simulink model "BatteryStoragePVPlantGFM"  (R2023a)
settings: Solver=FixedStepDiscrete  StartTime=0.0  StopTime=SimulationTime  RelTol=1e-3
PreLoadFcn:
  | run('BatteryStoragePVPlantGFMParameters')
undefined symbols (not defined in the file): Array, Base, battery, BatteryInverter, DiscIntNeverNeededParam, ee, Feeder, fRT, GFLBatteryController, GFMBatteryController, Grid, GridTransformer, Line, Load, Load2CB_final, Load2CB_initial, LVRT, maxSoC, maxVdc, minIrrad, minSoC, minVdc, Mpp, olTime, Panel, PVController, PVInverter, PVTransformer, Scenario, SM, SubTransmissionLine, Ts, VSMbase
libraries: ee_lib x51, nesl_utility x45, fl_lib x26, eeGeneralControl x18, simulink x12, eeTransforms x11, slpidlib x8, eePowerMeasurement x5, batteryecm_lib x2, eeTotalHarmonicDistorsion x2, spsLeadLagFilterLib x1, eeSmAC1C x1
(part 4 of 5)

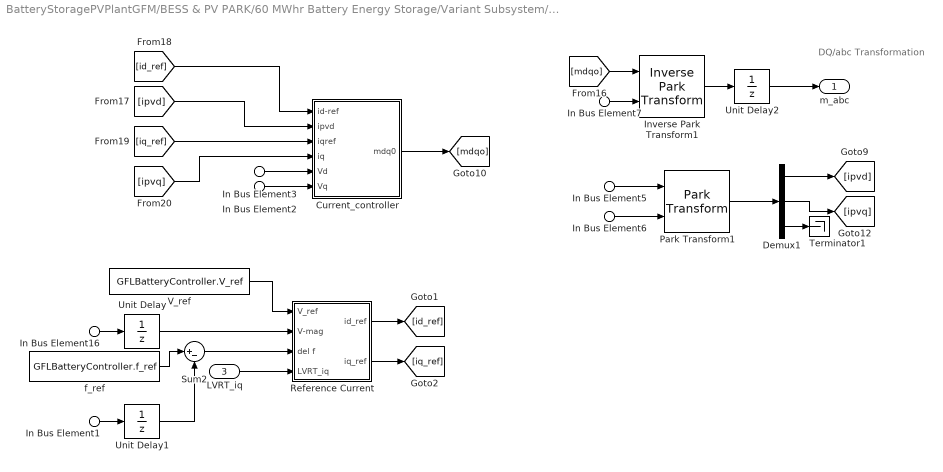
== system BatteryStoragePVPlantGFM/BESS & PV PARK/60 MWhr Battery Energy Storage/Variant Subsystem/Grid Following Support/Battery Inverter/GFL Battery Controller ==
  note: DQ/abc Transformation
  In Bus Element3 : Inport  PortName=Vbus  Element=Vd
  In Bus Element16 : Inport  PortName=Vbus  Element=Vd
  In Bus Element2 : Inport  PortName=Vbus  Element=Vq
  In Bus Element6 : Inport  PortName=Vbus  Element=Theta
  In Bus Element7 : Inport  PortName=Vbus  Element=Theta
  In Bus Element1 : Inport  PortName=Vbus  Element=w
  In Bus Element5 : Inport  Port=2  PortName=ipv2  Element=1
  LVRT_iq : Inport  Port=3
  Current_controller : Subsystem
  Demux1 : Demux  Outputs=3
  Inverse Park Transform1 : eeTransforms/Inverse Park Transform  AxisAlignment=Q-axis  PowerInvariant=off
  Park Transform1 : eeTransforms/Park Transform  AxisAlignment=Q-axis  PowerInvariant=off
  Reference Current : Subsystem
  Sum2 : Sum  Inputs=|+-
  Terminator1 : Terminator
  Unit Delay : UnitDelay  SampleTime=GFLBatteryController.Td  HasFrameUpgradeWarning=on
  Unit Delay1 : UnitDelay  SampleTime=GFLBatteryController.Td  HasFrameUpgradeWarning=on
  Unit Delay2 : UnitDelay  SampleTime=Ts  HasFrameUpgradeWarning=on
  V_ref : Constant  Value=GFLBatteryController.V_ref
  f_ref : Constant  Value=GFLBatteryController.f_ref
  m_abc : Outport
  wires:
  In Bus Element2/1 -> Current_controller/6(Vq)
  Current_controller/1(mdq0) -> [mdqo]
  Inverse Park Transform1/1 -> Unit Delay2/1
  Demux1/2 -> [ipvq]
  Unit Delay2/1 -> m_abc/1
  Demux1/1 -> [ipvd]
  Demux1/3 -> Terminator1/1
  [mdqo] -> Inverse Park Transform1/1
  Park Transform1/1 -> Demux1/1
  [id_ref] -> Current_controller/1(id-ref)
  In Bus Element3/1 -> Current_controller/5(Vd)
  [iq_ref] -> Current_controller/3(iqref)
  [ipvq] -> Current_controller/4(iq)
  In Bus Element6/1 -> Park Transform1/2
  In Bus Element7/1 -> Inverse Park Transform1/2
  [ipvd] -> Current_controller/2(ipvd)
  In Bus Element5/1 -> Park Transform1/1
  f_ref/1 -> Sum2/1
  V_ref/1 -> Reference Current/1(V_ref)
  In Bus Element16/1 -> Unit Delay/1
  LVRT_iq/1 -> Reference Current/4(LVRT_iq)
  Sum2/1 -> Reference Current/3(del f)
  Reference Current/2(iq_ref) -> [iq_ref]
  Reference Current/1(id_ref) -> [id_ref]
  In Bus Element1/1 -> Unit Delay1/1
  Unit Delay1/1 -> Sum2/2
  Unit Delay/1 -> Reference Current/2(V-mag)

== system BatteryStoragePVPlantGFM/BESS & PV PARK/60 MWhr Battery Energy Storage/Variant Subsystem/Grid Following Support/Battery Inverter/Inverter ==
  m_abc : Inport
  Average-Value Voltage Source Converter (Three-Phase) : ee_lib/Semiconductors & Converters/Converters/Average-Value Voltage Source Converter (Three-Phase)  port_option=ee.enum.threePhasePort.composite  frequency_option=ee.enum.converters.frequency.variable  FRated=60 Hz  losses_parameterization=ee.enum.converters.losses.fixed  Pfixed=1 W  ks=0.01  kc1=1.7 V  kc2=0.01 Ohm  Ploss_vect=[100, 800, 1870, 3250, 4900] W  Irms_vect=[10, 100, 200, 300, 400] A  Vdc_nom=300 V  thermal_mass=30000 J/K  temperature_specify=off  temperature_priority=High  temperature=298.15 K  temperature_nominal_specify=off  temperature_nominal_unit=K  temperature_nominal_value=1
      settings: InternalSimscapePortConfiguration="{\"Bottom\":[],\"Left\":[{\"id\":\"ModWave\",\"label\":\"ModWave\",\"type\":\"input\"},{\"id\":\"N\",\"label\":\"~\",\"type\":\"foundation.electrical.three_phase\"}],\"Right\":[{\"id\":\"p\",\"label\":\"+\",\"type\":\"foundation.electrical.electrical\"},{\"id\":\"n\",\"label\":\"-\",\"type\":\"foundation.electrical.electrical\"}],\"Top\":[]}"
  Average-Value DC-DC Converter : ee_lib/Semiconductors & Converters/Converters/Average-Value DC-DC Converter  control_option=ee.enum.converters.controlinput.voltage  converter_type=ee.enum.converters.dcdctype.buckboost  efficiency_option=ee.enum.converters.efficiency.constant  efficiency_fixed=99  i_vec=[0, 2, 5] A  efficiency_vec=[90, 95, 98]
      settings: InternalSimscapePortConfiguration="{\"Bottom\":[],\"Left\":[{\"id\":\"Vref\",\"label\":\"Vref\",\"type\":\"input\"},{\"id\":\"p1\",\"label\":\"1+\",\"type\":\"foundation.electrical.electrical\"},{\"id\":\"n1\",\"label\":\"1-\",\"type\":\"foundation.electrical.electrical\"}],\"Right\":[{\"id\":\"p2\",\"label\":\"2+\",\"type\":\"foundation.electrical.electrical\"},{\"id\":\"n2\",\"label\":\"2-\",\"type\":\"foundation.electrical.electrical\"}],\"Top\":[]}"
  Capacitor : fl_lib/Electrical/Electrical Elements/Capacitor  c=GFMBatteryController.C_dc F  r=1e-6 Ohm  g=0 1/Ohm  i_specify=off  i_priority=None  i=0 A  i_nominal_specify=off  i_nominal_unit=A  i_nominal_value=1  v_specify=off  v_priority=None  v=6560*.5 V  v_nominal_specify=off  v_nominal_unit=V  v_nominal_value=1  vc_specify=on  vc_priority=None  vc=PVInverter.Vdc V  vc_nominal_specify=off  vc_nominal_unit=V  vc_nominal_value=1
  Constant : Constant  Value=PVInverter.Vdc
  ERef1 : fl_lib/Electrical/Electrical Elements/Electrical Reference
  PS-Simulink Converter : nesl_utility/PS-Simulink Converter  PhysicalDomain=network_engine_domain  SubClassName=ps_output  LeftPortType=input  RightPortType=output  PseudoPeriodic=off  Frequencies=[]  VectorFormat=inherit  Unit=inherit  AffineConversion=off
  Simulink-PS Converter2 : nesl_utility/Simulink-PS Converter  PhysicalDomain=network_engine_domain  SubClassName=ps_input  LeftPortType=input  RightPortType=output  PseudoPeriodic=off  Frequencies=[]  NoiseDistribution=none  NoiseParameters=[]  Unit=1  AffineConversion=off  FilteringAndDerivatives=provide  SimscapeFilterOrder=1  InputFilterTimeConstant=0.001  UdotUserProvided=0
  Simulink-PS Converter3 : nesl_utility/Simulink-PS Converter  PhysicalDomain=network_engine_domain  SubClassName=ps_input  LeftPortType=input  RightPortType=output  PseudoPeriodic=off  Frequencies=[]  NoiseDistribution=none  NoiseParameters=[]  Unit=1  AffineConversion=off  FilteringAndDerivatives=provide  SimscapeFilterOrder=1  InputFilterTimeConstant=0.001  UdotUserProvided=0
  Unit Delay : UnitDelay  SampleTime=-1  HasFrameUpgradeWarning=on
  Voltage Sensor : fl_lib/Electrical/Electrical Sensors/Voltage Sensor
  battery : batteryecm_lib/Battery  Vnom=battery.vbat_nominal V  prm_dir=simscape.enum.battery.prm_dir.disabled  R1_dis=2 Ohm  R1_ch=2 Ohm  R1=battery.resistance Ohm  prm_AH=simscape.enum.battery.prm_AH.finite  AH=battery.capacity A*hr  V1=battery.vbat_1 V  AH1=battery.charge_vbat1 A*hr  prm_R2=simscape.enum.battery.prm_R2.disabled  R2=2000 Ohm  Tmeas=298.15 K  charge_measurement_port=simscape.enum.battery.enable.no  prm_dyn=simscape.enum.battery.prm_dyn.off  Rp1=0.005 Ohm  tau1=30 s  Rp2=0.005 Ohm  tau2=30 s  Rp3=0.005 Ohm  tau3=30 s  Rp4=0.005 Ohm  tau4=30 s  Rp5=0.005 Ohm  tau5=30 s  prm_fade=simscape.enum.battery.prm_fade.disabled  N_fade=100  AH_fade=45 A*hr  R1_fade=2.02 Ohm  R1_ch_fade=2.02 Ohm  V1_fade=10.35 V  prm_age=simscape.enum.battery.prm_age.disabled  prm_age_OCV=simscape.enum.battery.prm_age_OCV.OCV  OCV_age=0.9  SOC_age=60  Tmeas_age=298.15 K  delta_time_age_vec=[0] d  temperature_age_vec=[273] K  OCV_scaling_age=2.2134e6  OCV_offset_age=1.632e6  temp_exp_age=0.515833569 V  t_exp_age=0.75  Vnom_T2=12 V  R1_T2=2.2 Ohm  R1_T2_dis=2.2 Ohm  R1_T2_ch=2.2 Ohm  V1_T2=11.4 V  R2_T2=2200 Ohm  Rp1_T2=0.005 Ohm  tau1_T2=30 s  Rp2_T2=0.005 Ohm  tau2_T2=30 s  Rp3_T2=0.005 Ohm  tau3_T2=30 s  Rp4_T2=0.005 Ohm  tau4_T2=30 s  Rp5_T2=0.005 Ohm  tau5_T2=30 s  Tmeas2=273.15 K  thermal_port=simscape.enum.thermaleffects.omit  thermal_mass=30000 J/K  i_specify=off  i_priority=None  i=0 A  i_nominal_specify=off  i_nominal_unit=A  i_nominal_value=1  v_specify=on  v_priority=None  v=6000 V  v_nominal_specify=off  v_nominal_unit=V  v_nominal_value=1  charge_specify=off  charge_priority=High  charge=50 A*hr  charge_nominal_specify=off  charge_nominal_unit=A*hr  charge_nominal_value=1  num_cycles_specify=off  num_cycles_priority=High  num_cycles=0  num_cycles_nominal_specify=off  num_cycles_nominal_unit=1  num_cycles_nominal_value=1  temperature_specify=off  temperature_priority=High  temperature=298.15 K  temperature_nominal_specify=off  temperature_nominal_unit=K  temperature_nominal_value=1
  abc : PMIOPort  Side=Right
  wires:
  Constant/1 -> Unit Delay/1
  Unit Delay/1 -> Simulink-PS Converter3/1
  m_abc/1 -> Simulink-PS Converter2/1
  PS-Simulink Converter/1 -> [Vdc]
  connections:
  Average-Value DC-DC Converter/RConn2 -- ERef1/LConn1 -- Capacitor/RConn1 -- Average-Value Voltage Source Converter (Three-Phase)/RConn2 -- Voltage Sensor/RConn2
  Average-Value DC-DC Converter/RConn1 -- Capacitor/LConn1 -- Average-Value Voltage Source Converter (Three-Phase)/RConn1 -- Voltage Sensor/LConn1
  Simulink-PS Converter3/RConn1 -- Average-Value DC-DC Converter/LConn1
  Average-Value Voltage Source Converter (Three-Phase)/LConn1 -- Simulink-PS Converter2/RConn1
  battery/RConn1 -- Average-Value DC-DC Converter/LConn3
  battery/LConn1 -- Average-Value DC-DC Converter/LConn2
  PS-Simulink Converter/LConn1 -- Voltage Sensor/RConn1
  abc/RConn1 -- Average-Value Voltage Source Converter (Three-Phase)/LConn2

== system BatteryStoragePVPlantGFM/BESS & PV PARK/60 MWhr Battery Energy Storage/Variant Subsystem/Grid Forming VSM/Battery Inverter B1/Inverter ==
  note: DC bus voltage reference
  reference : Inport
  "Average DC_DC bidirectional Converter " : ee_lib/Semiconductors & Converters/Converters/Average-Value DC-DC Converter  control_option=ee.enum.converters.controlinput.voltage  converter_type=ee.enum.converters.dcdctype.buckboost  efficiency_option=ee.enum.converters.efficiency.constant  efficiency_fixed=99  i_vec=[0, 2, 5] A  efficiency_vec=[90, 95, 98]
      settings: InternalSimscapePortConfiguration="{\"Bottom\":[],\"Left\":[{\"id\":\"Vref\",\"label\":\"Vref\",\"type\":\"input\"},{\"id\":\"p1\",\"label\":\"1+\",\"type\":\"foundation.electrical.electrical\"},{\"id\":\"n1\",\"label\":\"1-\",\"type\":\"foundation.electrical.electrical\"}],\"Right\":[{\"id\":\"p2\",\"label\":\"2+\",\"type\":\"foundation.electrical.electrical\"},{\"id\":\"n2\",\"label\":\"2-\",\"type\":\"foundation.electrical.electrical\"}],\"Top\":[]}"
  Average-Value Voltage Source Inverter : ee_lib/Semiconductors & Converters/Converters/Average-Value Voltage Source Converter (Three-Phase)  port_option=ee.enum.threePhasePort.composite  frequency_option=ee.enum.converters.frequency.variable  FRated=60 Hz  losses_parameterization=ee.enum.converters.losses.fixed  Pfixed=0.1 W  ks=0.01  kc1=1.7 V  kc2=0.01 Ohm  Ploss_vect=[100, 800, 1870, 3250, 4900] W  Irms_vect=[10, 100, 200, 300, 400] A  Vdc_nom=300 V  thermal_mass=30000 J/K  temperature_specify=off  temperature_priority=High  temperature=298.15 K  temperature_nominal_specify=off  temperature_nominal_unit=K  temperature_nominal_value=1
      settings: InternalSimscapePortConfiguration="{\"Bottom\":[],\"Left\":[{\"id\":\"ModWave\",\"label\":\"ModWave\",\"type\":\"input\"},{\"id\":\"N\",\"label\":\"~\",\"type\":\"foundation.electrical.three_phase\"}],\"Right\":[{\"id\":\"p\",\"label\":\"+\",\"type\":\"foundation.electrical.electrical\"},{\"id\":\"n\",\"label\":\"-\",\"type\":\"foundation.electrical.electrical\"}],\"Top\":[]}"
  Battery (60MWhr) : batteryecm_lib/Battery  Vnom=battery.vbat_nominal V  prm_dir=simscape.enum.battery.prm_dir.disabled  R1_dis=2 Ohm  R1_ch=2 Ohm  R1=battery.resistance Ohm  prm_AH=simscape.enum.battery.prm_AH.finite  AH=battery.capacity A*hr  V1=battery.vbat_1 V  AH1=battery.charge_vbat1 A*hr  prm_R2=simscape.enum.battery.prm_R2.disabled  R2=2000 Ohm  Tmeas=298.15 K  charge_measurement_port=simscape.enum.battery.enable.no  prm_dyn=simscape.enum.battery.prm_dyn.off  Rp1=0.005 Ohm  tau1=30 s  Rp2=0.005 Ohm  tau2=30 s  Rp3=0.005 Ohm  tau3=30 s  Rp4=0.005 Ohm  tau4=30 s  Rp5=0.005 Ohm  tau5=30 s  prm_fade=simscape.enum.battery.prm_fade.disabled  N_fade=100  AH_fade=45 A*hr  R1_fade=2.02 Ohm  R1_ch_fade=2.02 Ohm  V1_fade=10.35 V  prm_age=simscape.enum.battery.prm_age.disabled  prm_age_OCV=simscape.enum.battery.prm_age_OCV.OCV  OCV_age=0.9  SOC_age=60  Tmeas_age=298.15 K  delta_time_age_vec=[0] d  temperature_age_vec=[273] K  OCV_scaling_age=2.2134e6  OCV_offset_age=1.632e6  temp_exp_age=0.515833569 V  t_exp_age=0.75  Vnom_T2=12 V  R1_T2=2.2 Ohm  R1_T2_dis=2.2 Ohm  R1_T2_ch=2.2 Ohm  V1_T2=11.4 V  R2_T2=2200 Ohm  Rp1_T2=0.005 Ohm  tau1_T2=30 s  Rp2_T2=0.005 Ohm  tau2_T2=30 s  Rp3_T2=0.005 Ohm  tau3_T2=30 s  Rp4_T2=0.005 Ohm  tau4_T2=30 s  Rp5_T2=0.005 Ohm  tau5_T2=30 s  Tmeas2=273.15 K  thermal_port=simscape.enum.thermaleffects.omit  thermal_mass=30000 J/K  i_specify=off  i_priority=None  i=0 A  i_nominal_specify=off  i_nominal_unit=A  i_nominal_value=1  v_specify=on  v_priority=None  v=6000 V  v_nominal_specify=off  v_nominal_unit=V  v_nominal_value=1  charge_specify=off  charge_priority=High  charge=50 A*hr  charge_nominal_specify=off  charge_nominal_unit=A*hr  charge_nominal_value=1  num_cycles_specify=off  num_cycles_priority=High  num_cycles=0  num_cycles_nominal_specify=off  num_cycles_nominal_unit=1  num_cycles_nominal_value=1  temperature_specify=off  temperature_priority=High  temperature=298.15 K  temperature_nominal_specify=off  temperature_nominal_unit=K  temperature_nominal_value=1
  Capacitor : fl_lib/Electrical/Electrical Elements/Capacitor  c=GFMBatteryController.C_dc F  r=1e-6 Ohm  g=0 1/Ohm  i_specify=off  i_priority=None  i=0 A  i_nominal_specify=off  i_nominal_unit=A  i_nominal_value=1  v_specify=off  v_priority=None  v=6560*.5 V  v_nominal_specify=off  v_nominal_unit=V  v_nominal_value=1  vc_specify=on  vc_priority=None  vc=PVInverter.Vdc V  vc_nominal_specify=off  vc_nominal_unit=V  vc_nominal_value=1
  Constant : Constant  Value=PVInverter.Vdc
  ERef1 : fl_lib/Electrical/Electrical Elements/Electrical Reference
  PS-Simulink Converter : nesl_utility/PS-Simulink Converter  PhysicalDomain=network_engine_domain  SubClassName=ps_output  LeftPortType=input  RightPortType=output  PseudoPeriodic=off  Frequencies=[]  VectorFormat=inherit  Unit=inherit  AffineConversion=off
  Simulink-PS Converter2 : nesl_utility/Simulink-PS Converter  PhysicalDomain=network_engine_domain  SubClassName=ps_input  LeftPortType=input  RightPortType=output  PseudoPeriodic=off  Frequencies=[]  NoiseDistribution=none  NoiseParameters=[]  Unit=1  AffineConversion=off  FilteringAndDerivatives=provide  SimscapeFilterOrder=1  InputFilterTimeConstant=0.001  UdotUserProvided=0
  Simulink-PS Converter3 : nesl_utility/Simulink-PS Converter  PhysicalDomain=network_engine_domain  SubClassName=ps_input  LeftPortType=input  RightPortType=output  PseudoPeriodic=off  Frequencies=[]  NoiseDistribution=none  NoiseParameters=[]  Unit=1  AffineConversion=off  FilteringAndDerivatives=provide  SimscapeFilterOrder=1  InputFilterTimeConstant=0.001  UdotUserProvided=0
  Unit Delay : UnitDelay  SampleTime=-1  HasFrameUpgradeWarning=on
  Voltage Sensor : fl_lib/Electrical/Electrical Sensors/Voltage Sensor
  abc : PMIOPort  Side=Right
  wires:
  PS-Simulink Converter/1 -> [Vdc]
  reference/1 -> Simulink-PS Converter2/1
  Unit Delay/1 -> Simulink-PS Converter3/1
  Constant/1 -> Unit Delay/1
  connections:
  PS-Simulink Converter/LConn1 -- Voltage Sensor/RConn1
  Capacitor/LConn1 -- Average-Value Voltage Source Inverter/RConn1 -- "Average DC_DC bidirectional Converter "/RConn1 -- Voltage Sensor/LConn1
  ERef1/LConn1 -- Capacitor/RConn1 -- Average-Value Voltage Source Inverter/RConn2 -- Voltage Sensor/RConn2 -- "Average DC_DC bidirectional Converter "/RConn2
  Average-Value Voltage Source Inverter/LConn1 -- Simulink-PS Converter2/RConn1
  abc/RConn1 -- Average-Value Voltage Source Inverter/LConn2
  Simulink-PS Converter3/RConn1 -- "Average DC_DC bidirectional Converter "/LConn1
  Battery (60MWhr)/LConn1 -- "Average DC_DC bidirectional Converter "/LConn2
  Battery (60MWhr)/RConn1 -- "Average DC_DC bidirectional Converter "/LConn3

== system BatteryStoragePVPlantGFM/BESS & PV PARK/60 MWhr Battery Energy Storage/Variant Subsystem/Grid Forming VSM/Battery Inverter B1/controller ==
  In Bus Element : Inport  PortName=Bat  Element=Iabc_bat
  In Bus Element1 : Inport  PortName=Bat  Element=Vabc_bat
  Constant : Constant  Value=GFMBatteryController.P_ref  SampleTime=Ts
  Constant1 : Constant  Value=GFMBatteryController.Q_ref  SampleTime=Ts
  GridFormingController : Subsystem  mask{power=VSMbase.power*1e3, girdLineVoltage=VSMbase.lineVoltage, powerFreq=VSMbase.frequency, powerControl=Virtual Synchronous Machine, activePowerSampleTime=GFMBatteryController.Sampletime, droopSlope=BatteryInverter.droopControl.freqSlopeMp, droopT1=BatteryInverter.droopControl.T1, droopT2=BatteryInverter.droopControl.T2, droopTC=BatteryInverter.droopControl.lpfTimeConst, vsmPmeasFilterTC=GFMBatteryController.filtertimeconstant, vsmFreqDroop=1/GFMBatteryController.frequencydroop, vsmInertiaTC=GFMBatteryController.VSMInertia, vsmDampingConst=GFMBatteryController.Damping, QVoltFilterTC=GFMBatteryController.reactivepowerfiltertimeconstant, QVoltDroop=GFMBatteryController.voltagedroop, currentLimit=Virtual Impedance, maxCurrentLimit=BatteryInverter.currentLimit.overNominalCurrent, ctLimitVirtualImp=BatteryInverter.currentLimit.virImpResistance, ctLimitXbyR=BatteryInverter.currentLimit.virImpXbyR, ctLimitMaxCurrent=BatteryInverter.currentLimit.currentIsdSaturationMax, ctLimitDelayTime=BatteryInverter.currentLimit.overCurrentIsdDelay, VdIGain=GFMBatteryController.voltagecontrolki, vdPGain=GFMBatteryController.voltagecontrolkp, voltControlTs=GFMBatteryController.voltagecontroltimeconstant, VdMaxCt=BatteryInverter.controller.VoltageMaxId, VdMinCt=BatteryInverter.controller.VoltageMinId, VqPGain=GFMBatteryController.voltagecontrolkp, VqIGain=GFMBatteryController.voltagecontrolki, VqMaxCt=BatteryInverter.controller.VoltageMaxIq, VqMinCt=BatteryInverter.controller.VoltageMinIq, dcBusVoltage=BatteryInverter.DCVoltage, filterInductance=BatteryInverter.L, currentControlTs=GFMBatteryController.currentcontrollersampletime, IdPGain=GFMBatteryController.currentcontrollerkp, IdIGain=GFMBatteryController.currentcontrollerki, IqPGain=GFMBatteryController.currentcontrollerkp, IqIGain=GFMBatteryController.currentcontrollerki}
      mask prompts: power "Gird power (kW)"; girdLineVoltage "Gird line voltage (V)"; powerFreq "Power frequency (Hz)"; powerControl "Active Power Control"; activePowerSampleTime "Sample time (s)"; droopSlope "Frequency droop slope (Hz/W)"; droopT1 "Lead-Lag Numerator time constant (s)"; droopT2 "Lead-Lag Denominator time constant (s)"; droopTC "Filter cut-off time constant (s)"; vsmPmeasFilterTC "P measurement filter time constant (s)"; vsmFreqDroop "Frequency droop gain"; vsmInertiaTC "Inertia time constant (s)"; vsmDampingConst "Damping constant (pu)"; QVoltFilterTC "Q measurement filter time constant (s)"; QVoltDroop "Voltage droop (pu)"; currentLimit "Current Limiting Method"; maxCurrentLimit "Current Limit (pu)"; ctLimitVirtualImp "Virtual impedance (pu)"; ctLimitXbyR "Virtual X/R ratio"; ctLimitMaxCurrent "Maximum allowed current (pu)"; ctLimitDelayTime "Max. current delay time (s)"; VdIGain "Vd integral gain"; vdPGain "Vd proportaion gain"; voltControlTs "Controller sample time (s)"; VdMaxCt "Vd max. current Limit (A)"; VdMinCt "Vd min. current Limit (A)"; VqPGain "Vq proportaion gain"; VqIGain "Vq integration gain"; VqMaxCt "Vq max. current Limit (A)"; VqMinCt "Vq min. current Limit (A)"; dcBusVoltage "DC bus voltage"; filterInductance "Filter inductance (H)"; currentControlTs "Controller sample time (s)"; IdPGain "Id proportaion gain"; IdIGain "Id integral gain"; IqPGain "Iq proportaion gain"; IqIGain "Iq integral gain"
      mask init:
      | powerChoice = get_param(gcb,'powerControl');
      | currentChoice = get_param(gcb,'currentLimit');
      | 
      | powerloc = [gcb, '/Power Control/ActivePowerControl']; 
      | currentloc = [gcb, '/Current Limiting/CurrentLimitingMethod'];
      | 
      | switch powerChoice
      |     case 'Virtual Synchronous Machine'
      |         set_param(powerloc, 'LabelModeActiveChoice', 'vsm');
      |     case 'Droop Control'
      |          set_param(powerloc, 'LabelModeActiveChoice', 'droop');
      |    otherwise
      |         disp('Choose proper active power control method')
      | end
      | switch currentChoice
      |     case 'Virtual Impedance'
      |           set_param(currentloc, 'LabelModeActiveChoice', 'virimp');
      |     case 'Current Limiting'
      |          set_param(currentloc, 'LabelModeActiveChoice', 'ctSat');
      |     case 'Both Virtual Impedance and Current Limiting'
      |             set_param(currentloc, 'LabelModeActiveChoice', 'both');
      |     otherwise
      |         disp('Choose proper current limiting method')
      | end
      mask TypeOptions powerControl: Virtual Synchronous Machine | Droop Control
      mask Callback powerControl:
      | h = Simulink.Mask.get(gcb);
      | slectedActivePowerControl=get_param(gcb,'powerControl');
      | %slectedActivePowerControl = h.Parameters(find(string({h.Parameters.Name}) == 'powerControl')).Value;
      | switch slectedActivePowerControl
      |     case 'Virtual Synchronous Machine'
      |         h.Parameters(find(string({h.Parameters.Name}) == 'droopSlope')).Visible = 'off';
      |         h.Parameters(find(string({h.Parameters.Name}) == 'droopTC')).Visible = 'off';
      |         h.Parameters(find(string({h.Parameters.Name}) == 'droopT1')).Visible = 'off';
      |         h.Parameters(find(string({h.Parameters.Name}) == 'droopT2')).Visible = 'off';
      |         h.Parameters(find(string({h.Parameters.Name}) == 'vsmPmeasFilterTC')).Visible = 'on';
      |         h.Parameters(find(string({h.Parameters.Name}) == 'vsmFreqDroop')).Visible = 'on';
      |         h.Parameters(find(string({h.Parameters.Name}) == 'vsmInertiaTC')).Visible = 'on';
      |         h.Parameters(find(string({h.Parameters.Name}) == 'vsmDampingConst')).Visible = 'on';
      |     case 'Droop Control'
      |         h.Parameters(find(string({h.Parameters.Name}) == 'droopSlope')).Visible = 'on';
      |         h.Parameters(find(string({h.Parameters.Name}) == 'droopTC')).Visible = 'on';
      |         h.Parameters(find(string({h.Parameters.Name}) == 'droopT1')).Visible = 'on';
      |         h.Parameters(find(string({h.Parameters.Name}) == 'droopT2')).Visible = 'on';
      |         h.Parameters(find(string({h.Parameters.Name}) == 'vsmPmeasFilterTC')).Visible = 'off';
      |         h.Parameters(find(string({h.Parameters.Name}) == 'vsmFreqDroop')).Visible = 'off';
      |         h.Parameters(find(string({h.Parameters.Name}) == 'vsmInertiaTC')).Visible = 'off';
      |         h.Parameters(find(string({h.Parameters.Name}) == 'vsmDampingConst')).Visible = 'off';
      |     otherwise
      |         disp('Choose proper active power control method')
      | end
      mask TypeOptions currentLimit: Virtual Impedance | Current Limiting
      mask Callback currentLimit:
      | currentLimit = 1;
      | h = Simulink.Mask.get(gcb);
      | currentLimitControl=get_param(gcb,'currentLimit');
      | %slectedActivePowerControl = h.Parameters(find(string({h.Parameters.Name}) == 'powerControl')).Value;
      | switch currentLimitControl
      |     case 'Virtual Impedance'
      |         h.Parameters(find(string({h.Parameters.Name}) == 'maxCurrentLimit')).Visible = 'on';
      |         h.Parameters(find(string({h.Parameters.Name}) == 'ctLimitVirtualImp')).Visible = 'on';
      |         h.Parameters(find(string({h.Parameters.Name}) == 'ctLimitXbyR')).Visible = 'on';
      |         h.Parameters(find(string({h.Parameters.Name}) == 'ctLimitMaxCurrent')).Visible = 'off';
      |         h.Parameters(find(string({h.Parameters.Name}) == 'ctLimitDelayTime')).Visible = 'off';
      |     case 'Current Limiting'
      |         h.Parameters(find(string({h.Parameters.Name}) == 'maxCurrentLimit')).Visible = 'off';
      |         h.Parameters(find(string({h.Parameters.Name}) == 'ctLimitVirtualImp')).Visible = 'off';
      |         h.Parameters(find(string({h.Parameters.Name}) == 'ctLimitXbyR')).Visible = 'off';
      |         h.Parameters(find(string({h.Parameters.Name}) == 'ctLimitMaxCurrent')).Visible = 'on';
      |         h.Parameters(find(string({h.Parameters.Name}) == 'ctLimitDelayTime')).Visible = 'on';
      |     case 'Both Virtual Impedance and Current Limiting'
      |         h.Parameters(find(string({h.Parameters.Name}) == 'maxCurrentLimit')).Visible = 'on';
      |         h.Parameters(find(string({h.Parameters.Name}) == 'ctLimitVirtualImp')).Visible = 'on';
      |         h.Parameters(find(string({h.Parameters.Name}) == 'ctLimitXbyR')).Visible = 'on';
      |         h.Parameters(find(string({h.Parameters.Name}) == 'ctLimitMaxCurrent')).Visible = 'on';
      |         h.Parameters(find(string({h.Parameters.Name}) == 'ctLimitDelayTime')).Visible = 'on';
      |     otherwise
      |         disp('Choose proper current limiting method')
      | end
      mask DialogControl Container8 Prompt: Grid-forming inverter parameters
      mask DialogControl Pcontrolgrp Prompt: Active Power Controller Parameters
      mask DialogControl QcontrolGrp Prompt: Reactive Power Controller Parameters
      mask DialogControl faultRideThroughGrp Prompt: Fault Ride Through Parameters
      mask DialogControl voltControlgrp Prompt: Voltage Controller Parameters
      mask DialogControl Container15currentContGrp Prompt: Current Controller Parameters
      mask Display: image('C:\Users\rajarshd\OneDrive - MathWorks\Simulation_Final\Pics\e_vsm.png'); % Use "Edit Image" on toolstrip to change.
  Unit Delay2 : UnitDelay  SampleTime=Ts  HasFrameUpgradeWarning=on
  mabc : Outport
  wires:
  GridFormingController/2(Pmeas) -> [Pmeas]
  GridFormingController/3(Qmeas) -> [Qmeas]
  Constant1/1 -> GridFormingController/2(Qref)
  GridFormingController/1(mabc) -> Unit Delay2/1
  Constant/1 -> GridFormingController/1(Pref)
  Unit Delay2/1 -> mabc/1
  In Bus Element/1 -> GridFormingController/3(Igabc)
  In Bus Element1/1 -> GridFormingController/4(Vgabc)

== system BatteryStoragePVPlantGFM/BESS & PV PARK/100 MWp PV Park/PV Inverter A1/PV Controller/DC voltage controller & current reference/Subsystem1/V_dc_Controller1 ==
  PV_plant1 : Inport
  In2 : Inport  Port=2
  Gain : Gain  Gain=1/PVController.Vdc_base
  PID Controller : slpidlib/PID Controller  Controller=PID  Form=Parallel  TimeDomain=Discrete-time  UseExternalTs=off  SampleTime=-1  IntegratorMethod=Forward Euler  FilterMethod=Forward Euler  ControllerParametersSource=internal  P=PVController.Kp_v  I=PVController.Ki_v  UseKiTs=off  D=PVController.Kd_v  N=100  UseFilter=on  TunerSelectOption=Transfer Function Based (PID Tuner App)  ZeroCross=off  InitialConditionSource=internal  InitialConditionForIntegrator=0  InitialConditionForFilter=0  DifferentiatorICPrevScaledInput=0  ExternalReset=none  TrackingMode=off  Kt=1  LimitOutput=off  SatLimitsSource=internal  UpperSaturationLimit=inf  LowerSaturationLimit=-inf  LinearizeAsGain=on  AntiWindupMode=none  Kb=1  LimitIntegrator=off  UpperIntegratorSaturationLimit=inf  LowerIntegratorSaturationLimit=-inf  POutMin=[]  POutMax=[]  IOutMin=[]  IOutMax=[]  DOutMin=[]  DOutMax=[]  NOutMin=[]  NOutMax=[]  SumOutMin=[]  SumOutMax=[]  SaturationOutMin=[]  SaturationOutMax=[]  PParamMin=[]  PParamMax=[]  IParamMin=[]  IParamMax=[]  DParamMin=[]  DParamMax=[]  NParamMin=[]  NParamMax=[]  KbParamMin=[]  KbParamMax=[]  KtParamMin=[]  KtParamMax=[]  KbOutMin=[]  KbOutMax=[]  KtOutMin=[]  KtOutMax=[]  IntegratorOutMin=[]  IntegratorOutMax=[]  FilterOutMin=[]  FilterOutMax=[]  SumI1OutMin=[]  SumI1OutMax=[]  SumI2OutMin=[]  SumI2OutMax=[]  SumI3OutMin=[]  SumI3OutMax=[]  SumI4OutMin=[]  SumI4OutMax=[]  SumDOutMin=[]  SumDOutMax=[]  DifferentiatorOutMin=[]  DifferentiatorOutMax=[]  FilterDiffOutCoefMin=[]  FilterDiffOutCoefMax=[]  ReciprocalOutMin=[]  ReciprocalOutMax=[]  SumDenOutMin=[]  SumDenOutMax=[]  SumNumOutMin=[]  SumNumOutMax=[]  DivideOutMin=[]  DivideOutMax=[]  UdiffTsProdOutMin=[]  UdiffTsProdOutMax=[]  NTsProdOutMin=[]  NTsProdOutMax=[]  UintegralTsProdOutMin=[]  UintegralTsProdOutMax=[]  UngainTsProdOutMin=[]  UngainTsProdOutMax=[]  ClampingZeroOutDataTypeStr=Inherit: Inherit via back propagation  ClampingZeroOutMin=[]  ClampingZeroOutMax=[]  FilterDenConstantOutDataTypeStr=Inherit: Inherit via back propagation  FilterDenConstantOutMin=[]  FilterDenConstantOutMax=[]  PCopyOutDataTypeStr=Inherit: Inherit via back propagation  PCopyOutMin=[]  PCopyOutMax=[]  NCopyOutDataTypeStr=Inherit: Inherit via back propagation  NCopyOutMin=[]  NCopyOutMax=[]  IntegratorContinuousStateAttributes=''  IntegratorStateMustResolveToSignalObject=off  IntegratorRTWStateStorageClass=Auto  FilterContinuousStateAttributes=''  FilterStateMustResolveToSignalObject=off  FilterRTWStateStorageClass=Auto  ParallelPVariant=InternalParameters  IdealPVariant=Disabled  IVariant=InternalParameters  DVariant=InternalParameters  IntegratorVariant=Discrete  SatVariant=Disabled  AWVariant=Passthrough  PCopyVariant=Disabled  TRVariant=Disabled  FdbkBlocksVariant=Forward  IdealPFdbkVariant=Disabled  SatFdbkVariant=Disabled  DerivativeFilterVariant=ForwardEulerFilter  NVariant=InternalParameters  NCopyVariant=Disabled  FilterICVariant=InternalICsFilter  IntegratorICVariant=InternalICs  ExternalResetVariant=Disabled  TRSumVariant=Passthrough  SumFdbkVariant=Disabled  SumVariant=Sum_PID  TsampFilterVariant=InternalTs  TsampNgainVariant=Passthrough  TsampIntegralVariant=Disabled_SignalSpec  ExternalSaturationOutDataTypeStr=Inherit: Same as second input
  Sum : Sum  Inputs=|+-
  Out1 : Outport
  wires:
  PV_plant1/1 -> Sum/1
  In2/1 -> Sum/2
  PID Controller/1 -> Out1/1
  Gain/1 -> PID Controller/1
  Sum/1 -> Gain/1

== system BatteryStoragePVPlantGFM/BESS & PV PARK/100 MWp PV Park/PV Inverter A2/PV Controller/DC voltage controller & current reference/Subsystem1/V_dc_Controller1 ==
  PV_plant1 : Inport
  In2 : Inport  Port=2
  Gain : Gain  Gain=1/PVController.Vdc_base
  PID Controller : slpidlib/PID Controller  Controller=PID  Form=Parallel  TimeDomain=Discrete-time  UseExternalTs=off  SampleTime=-1  IntegratorMethod=Forward Euler  FilterMethod=Forward Euler  ControllerParametersSource=internal  P=PVController.Kp_v  I=PVController.Ki_v  UseKiTs=off  D=PVController.Kd_v  N=100  UseFilter=on  TunerSelectOption=Transfer Function Based (PID Tuner App)  ZeroCross=off  InitialConditionSource=internal  InitialConditionForIntegrator=0  InitialConditionForFilter=0  DifferentiatorICPrevScaledInput=0  ExternalReset=none  TrackingMode=off  Kt=1  LimitOutput=off  SatLimitsSource=internal  UpperSaturationLimit=inf  LowerSaturationLimit=-inf  LinearizeAsGain=on  AntiWindupMode=none  Kb=1  LimitIntegrator=off  UpperIntegratorSaturationLimit=inf  LowerIntegratorSaturationLimit=-inf  POutMin=[]  POutMax=[]  IOutMin=[]  IOutMax=[]  DOutMin=[]  DOutMax=[]  NOutMin=[]  NOutMax=[]  SumOutMin=[]  SumOutMax=[]  SaturationOutMin=[]  SaturationOutMax=[]  PParamMin=[]  PParamMax=[]  IParamMin=[]  IParamMax=[]  DParamMin=[]  DParamMax=[]  NParamMin=[]  NParamMax=[]  KbParamMin=[]  KbParamMax=[]  KtParamMin=[]  KtParamMax=[]  KbOutMin=[]  KbOutMax=[]  KtOutMin=[]  KtOutMax=[]  IntegratorOutMin=[]  IntegratorOutMax=[]  FilterOutMin=[]  FilterOutMax=[]  SumI1OutMin=[]  SumI1OutMax=[]  SumI2OutMin=[]  SumI2OutMax=[]  SumI3OutMin=[]  SumI3OutMax=[]  SumI4OutMin=[]  SumI4OutMax=[]  SumDOutMin=[]  SumDOutMax=[]  DifferentiatorOutMin=[]  DifferentiatorOutMax=[]  FilterDiffOutCoefMin=[]  FilterDiffOutCoefMax=[]  ReciprocalOutMin=[]  ReciprocalOutMax=[]  SumDenOutMin=[]  SumDenOutMax=[]  SumNumOutMin=[]  SumNumOutMax=[]  DivideOutMin=[]  DivideOutMax=[]  UdiffTsProdOutMin=[]  UdiffTsProdOutMax=[]  NTsProdOutMin=[]  NTsProdOutMax=[]  UintegralTsProdOutMin=[]  UintegralTsProdOutMax=[]  UngainTsProdOutMin=[]  UngainTsProdOutMax=[]  ClampingZeroOutDataTypeStr=Inherit: Inherit via back propagation  ClampingZeroOutMin=[]  ClampingZeroOutMax=[]  FilterDenConstantOutDataTypeStr=Inherit: Inherit via back propagation  FilterDenConstantOutMin=[]  FilterDenConstantOutMax=[]  PCopyOutDataTypeStr=Inherit: Inherit via back propagation  PCopyOutMin=[]  PCopyOutMax=[]  NCopyOutDataTypeStr=Inherit: Inherit via back propagation  NCopyOutMin=[]  NCopyOutMax=[]  IntegratorContinuousStateAttributes=''  IntegratorStateMustResolveToSignalObject=off  IntegratorRTWStateStorageClass=Auto  FilterContinuousStateAttributes=''  FilterStateMustResolveToSignalObject=off  FilterRTWStateStorageClass=Auto  ParallelPVariant=InternalParameters  IdealPVariant=Disabled  IVariant=InternalParameters  DVariant=InternalParameters  IntegratorVariant=Discrete  SatVariant=Disabled  AWVariant=Passthrough  PCopyVariant=Disabled  TRVariant=Disabled  FdbkBlocksVariant=Forward  IdealPFdbkVariant=Disabled  SatFdbkVariant=Disabled  DerivativeFilterVariant=ForwardEulerFilter  NVariant=InternalParameters  NCopyVariant=Disabled  FilterICVariant=InternalICsFilter  IntegratorICVariant=InternalICs  ExternalResetVariant=Disabled  TRSumVariant=Passthrough  SumFdbkVariant=Disabled  SumVariant=Sum_PID  TsampFilterVariant=InternalTs  TsampNgainVariant=Passthrough  TsampIntegralVariant=Disabled_SignalSpec  ExternalSaturationOutDataTypeStr=Inherit: Same as second input
  Sum : Sum  Inputs=|+-
  Out1 : Outport
  wires:
  PV_plant1/1 -> Sum/1
  In2/1 -> Sum/2
  PID Controller/1 -> Out1/1
  Gain/1 -> PID Controller/1
  Sum/1 -> Gain/1

== system BatteryStoragePVPlantGFM/BESS & PV PARK/60 MWhr Battery Energy Storage/Variant Subsystem/Grid Following Support/Battery Inverter/GFL Battery Controller/Current_controller ==
  id-ref : Inport
  ipvd : Inport  Port=2
  iqref : Inport  Port=3
  iq : Inport  Port=4
  Vd : Inport  Port=5
  Vq : Inport  Port=6
  Constant4 : Constant  Value=0
  Gain1 : Gain  Gain=2*1*pi*60*PVInverter.L/Base.z_base
  Gain2 : Gain  Gain=2*1*pi*60*PVInverter.L/Base.z_base
  Mux1 : Mux  Inputs=3
  PID Controller : slpidlib/PID Controller  Controller=PID  Form=Parallel  TimeDomain=Discrete-time  UseExternalTs=off  SampleTime=-1  IntegratorMethod=Forward Euler  FilterMethod=Forward Euler  ControllerParametersSource=internal  P=PVController.Kp_ic  I=PVController.Ki_ic  UseKiTs=off  D=PVController.Kd  N=100  UseFilter=on  TunerSelectOption=Transfer Function Based (PID Tuner App)  InitialConditionSource=internal  InitialConditionForIntegrator=0  InitialConditionForFilter=0  DifferentiatorICPrevScaledInput=0  ExternalReset=none  TrackingMode=off  Kt=1  LimitOutput=off  SatLimitsSource=internal  UpperSaturationLimit=inf  LowerSaturationLimit=-inf  LinearizeAsGain=on  AntiWindupMode=none  Kb=1  LimitIntegrator=off  UpperIntegratorSaturationLimit=inf  LowerIntegratorSaturationLimit=-inf  POutMin=[]  POutMax=[]  IOutMin=[]  IOutMax=[]  DOutMin=[]  DOutMax=[]  NOutMin=[]  NOutMax=[]  SumOutMin=[]  SumOutMax=[]  SaturationOutMin=[]  SaturationOutMax=[]  PParamMin=[]  PParamMax=[]  IParamMin=[]  IParamMax=[]  DParamMin=[]  DParamMax=[]  NParamMin=[]  NParamMax=[]  KbParamMin=[]  KbParamMax=[]  KtParamMin=[]  KtParamMax=[]  KbOutMin=[]  KbOutMax=[]  KtOutMin=[]  KtOutMax=[]  IntegratorOutMin=[]  IntegratorOutMax=[]  FilterOutMin=[]  FilterOutMax=[]  SumI1OutMin=[]  SumI1OutMax=[]  SumI2OutMin=[]  SumI2OutMax=[]  SumI3OutMin=[]  SumI3OutMax=[]  SumI4OutMin=[]  SumI4OutMax=[]  SumDOutMin=[]  SumDOutMax=[]  DifferentiatorOutMin=[]  DifferentiatorOutMax=[]  FilterDiffOutCoefMin=[]  FilterDiffOutCoefMax=[]  ReciprocalOutMin=[]  ReciprocalOutMax=[]  SumDenOutMin=[]  SumDenOutMax=[]  SumNumOutMin=[]  SumNumOutMax=[]  DivideOutMin=[]  DivideOutMax=[]  UdiffTsProdOutMin=[]  UdiffTsProdOutMax=[]  NTsProdOutMin=[]  NTsProdOutMax=[]  UintegralTsProdOutMin=[]  UintegralTsProdOutMax=[]  UngainTsProdOutMin=[]  UngainTsProdOutMax=[]  ClampingZeroOutDataTypeStr=Inherit: Inherit via back propagation  ClampingZeroOutMin=[]  ClampingZeroOutMax=[]  FilterDenConstantOutDataTypeStr=Inherit: Inherit via back propagation  FilterDenConstantOutMin=[]  FilterDenConstantOutMax=[]  PCopyOutDataTypeStr=Inherit: Inherit via back propagation  PCopyOutMin=[]  PCopyOutMax=[]  NCopyOutDataTypeStr=Inherit: Inherit via back propagation  NCopyOutMin=[]  NCopyOutMax=[]  IntegratorContinuousStateAttributes=''  IntegratorStateMustResolveToSignalObject=off  IntegratorRTWStateStorageClass=Auto  FilterContinuousStateAttributes=''  FilterStateMustResolveToSignalObject=off  FilterRTWStateStorageClass=Auto  ParallelPVariant=InternalParameters  IdealPVariant=Disabled  IVariant=InternalParameters  DVariant=InternalParameters  IntegratorVariant=Discrete  SatVariant=Disabled  AWVariant=Passthrough  PCopyVariant=Disabled  TRVariant=Disabled  FdbkBlocksVariant=Forward  IdealPFdbkVariant=Disabled  SatFdbkVariant=Disabled  DerivativeFilterVariant=ForwardEulerFilter  NVariant=InternalParameters  NCopyVariant=Disabled  FilterICVariant=InternalICsFilter  IntegratorICVariant=InternalICs  ExternalResetVariant=Disabled  TRSumVariant=Passthrough  SumFdbkVariant=Disabled  SumVariant=Sum_PID  TsampFilterVariant=InternalTs  TsampNgainVariant=Passthrough  TsampIntegralVariant=Disabled_SignalSpec  ExternalSaturationOutDataTypeStr=Inherit: Same as second input
  PID Controller1 : slpidlib/PID Controller  Controller=PID  Form=Parallel  TimeDomain=Discrete-time  UseExternalTs=off  SampleTime=-1  IntegratorMethod=Forward Euler  FilterMethod=Forward Euler  ControllerParametersSource=internal  P=PVController.Kp_ic  I=PVController.Ki_ic  UseKiTs=off  D=PVController.Kd  N=100  UseFilter=on  TunerSelectOption=Transfer Function Based (PID Tuner App)  InitialConditionSource=internal  InitialConditionForIntegrator=0  InitialConditionForFilter=0  DifferentiatorICPrevScaledInput=0  ExternalReset=none  TrackingMode=off  Kt=1  LimitOutput=off  SatLimitsSource=internal  UpperSaturationLimit=inf  LowerSaturationLimit=-inf  LinearizeAsGain=on  AntiWindupMode=none  Kb=1  LimitIntegrator=off  UpperIntegratorSaturationLimit=inf  LowerIntegratorSaturationLimit=-inf  POutMin=[]  POutMax=[]  IOutMin=[]  IOutMax=[]  DOutMin=[]  DOutMax=[]  NOutMin=[]  NOutMax=[]  SumOutMin=[]  SumOutMax=[]  SaturationOutMin=[]  SaturationOutMax=[]  PParamMin=[]  PParamMax=[]  IParamMin=[]  IParamMax=[]  DParamMin=[]  DParamMax=[]  NParamMin=[]  NParamMax=[]  KbParamMin=[]  KbParamMax=[]  KtParamMin=[]  KtParamMax=[]  KbOutMin=[]  KbOutMax=[]  KtOutMin=[]  KtOutMax=[]  IntegratorOutMin=[]  IntegratorOutMax=[]  FilterOutMin=[]  FilterOutMax=[]  SumI1OutMin=[]  SumI1OutMax=[]  SumI2OutMin=[]  SumI2OutMax=[]  SumI3OutMin=[]  SumI3OutMax=[]  SumI4OutMin=[]  SumI4OutMax=[]  SumDOutMin=[]  SumDOutMax=[]  DifferentiatorOutMin=[]  DifferentiatorOutMax=[]  FilterDiffOutCoefMin=[]  FilterDiffOutCoefMax=[]  ReciprocalOutMin=[]  ReciprocalOutMax=[]  SumDenOutMin=[]  SumDenOutMax=[]  SumNumOutMin=[]  SumNumOutMax=[]  DivideOutMin=[]  DivideOutMax=[]  UdiffTsProdOutMin=[]  UdiffTsProdOutMax=[]  NTsProdOutMin=[]  NTsProdOutMax=[]  UintegralTsProdOutMin=[]  UintegralTsProdOutMax=[]  UngainTsProdOutMin=[]  UngainTsProdOutMax=[]  ClampingZeroOutDataTypeStr=Inherit: Inherit via back propagation  ClampingZeroOutMin=[]  ClampingZeroOutMax=[]  FilterDenConstantOutDataTypeStr=Inherit: Inherit via back propagation  FilterDenConstantOutMin=[]  FilterDenConstantOutMax=[]  PCopyOutDataTypeStr=Inherit: Inherit via back propagation  PCopyOutMin=[]  PCopyOutMax=[]  NCopyOutDataTypeStr=Inherit: Inherit via back propagation  NCopyOutMin=[]  NCopyOutMax=[]  IntegratorContinuousStateAttributes=''  IntegratorStateMustResolveToSignalObject=off  IntegratorRTWStateStorageClass=Auto  FilterContinuousStateAttributes=''  FilterStateMustResolveToSignalObject=off  FilterRTWStateStorageClass=Auto  ParallelPVariant=InternalParameters  IdealPVariant=Disabled  IVariant=InternalParameters  DVariant=InternalParameters  IntegratorVariant=Discrete  SatVariant=Disabled  AWVariant=Passthrough  PCopyVariant=Disabled  TRVariant=Disabled  FdbkBlocksVariant=Forward  IdealPFdbkVariant=Disabled  SatFdbkVariant=Disabled  DerivativeFilterVariant=ForwardEulerFilter  NVariant=InternalParameters  NCopyVariant=Disabled  FilterICVariant=InternalICsFilter  IntegratorICVariant=InternalICs  ExternalResetVariant=Disabled  TRSumVariant=Passthrough  SumFdbkVariant=Disabled  SumVariant=Sum_PID  TsampFilterVariant=InternalTs  TsampNgainVariant=Passthrough  TsampIntegralVariant=Disabled_SignalSpec  ExternalSaturationOutDataTypeStr=Inherit: Same as second input
  Sum1 : Sum  Inputs=|+-
  Sum3 : Sum  Inputs=|++-
  Sum4 : Sum  Inputs=|+++
  Sum5 : Sum  Inputs=|+-
  mdq0 : Outport
  wires:
  PID Controller/1 -> Sum3/2
  Sum3/1 -> Mux1/1, [Ed]
  Gain2/1 -> Sum3/3
  ipvd/1 -> Gain1/1, Sum1/2
  id-ref/1 -> Sum1/1
  Gain1/1 -> Sum4/3
  Vq/1 -> Sum4/2
  iq/1 -> Gain2/1, Sum5/2
  Sum1/1 -> PID Controller/1
  Vd/1 -> Sum3/1
  Constant4/1 -> Mux1/3
  Sum5/1 -> PID Controller1/1
  iqref/1 -> Sum5/1
  PID Controller1/1 -> Sum4/1
  Sum4/1 -> Mux1/2, [Eq]
  Mux1/1 -> mdq0/1

== system BatteryStoragePVPlantGFM/BESS & PV PARK/60 MWhr Battery Energy Storage/Variant Subsystem/Grid Following Support/Battery Inverter/GFL Battery Controller/Reference Current ==
  note: Refernce Generation
  note: Current Limiters
  note: Avoid division by zero during start
  V_ref : Inport
  V-mag : Inport  Port=2
  del f : Inport  Port=3
  LVRT_iq : Inport  Port=4
  Constant : Constant  Value=GFLBatteryController.Q_ref
  Constant1 : Constant
  Constant3 : Constant  Value=PVInverter.I_max_pu
  Current limits : Subsystem
  Refernce id generation : Subsystem
  Refernce iq generation : Subsystem
  Switch : Switch  Criteria=u2 ~= 0  SaturateOnIntegerOverflow=off  InputSameDT=off
  Unit Delay1 : UnitDelay  SampleTime=Ts  HasFrameUpgradeWarning=on
  Unit Delay3 : UnitDelay  SampleTime=Ts  HasFrameUpgradeWarning=on
  id_ref : Outport
  iq_ref : Outport  Port=2
  wires:
  Current limits/1(iubd) -> [ubid]
  Unit Delay1/1 -> Current limits/2(iqref)
  Current limits/2(iubq) -> [ubiq]
  Unit Delay3/1 -> Current limits/3(idref)
  Constant3/1 -> Current limits/1(Imax)
  Refernce id generation/1(id_ref) -> id_ref/1, Unit Delay3/1
  del f/1 -> Refernce id generation/2(del f)
  V_ref/1 -> Refernce iq generation/1(V_ref)
  Refernce iq generation/1(iq_ref) -> Unit Delay1/1, iq_ref/1
  LVRT_iq/1 -> Refernce iq generation/3(LVRT_iq)
  [ubiq] -> Refernce iq generation/4(ubiq)
  [ubid] -> Refernce id generation/3(ubid)
  V-mag/1 -> Switch/1, Switch/2
  Switch/1 -> Refernce id generation/1(V_mag), Refernce iq generation/2(V_mag)
  Constant1/1 -> Switch/3
  Constant/1 -> Refernce iq generation/5(Q_ref)

== system BatteryStoragePVPlantGFM/BESS & PV PARK/60 MWhr Battery Energy Storage/Variant Subsystem/Grid Forming VSM/Battery Inverter B1/controller/GridFormingController ==
  Pref : Inport
  Qref : Inport  Port=2
  Igabc : Inport  Port=3
  Vgabc : Inport  Port=4
  Current Limiting : Subsystem
  Measurement : Subsystem
  Power Control : Subsystem
  VoltageCurrentControl : Subsystem
      settings: PortSchema="{\"entries\":[{\"content\":{\"sides\":[{\"content\":{\"connectorIds\":[\"In1\",\"In2\"]},\"type\":\"ConnectorPlacement.EquallySpacedRectSide\",\"uuid\":\"0bf15a12-7bc0-47e4-89bd-435769673763\"},{\"content\":{\"connectorIds\":[\"Out1\"],\"side\":\"RIGHT\"},\"type\":\"ConnectorPlacement.EquallySpacedRectSide\",\"uuid\":\"44a15d74-8878-4ec6-abe4-be0b1b609519\"},{\"content\":{\"connectorIds\":[\"In3\"],\"side\":\"TOP\"},\"type\":\"ConnectorPlacement.EquallySpacedRectSide\",\"uuid\":\"7a96781e-5638-4b2a-8101-d5785aae9f0f\"}]},\"type\":\"ConnectorPlacement.EquallySpacedConnector\",\"uuid\":\"4b3373ad-cf20-4175-894e-3bd1604dd0ce\"}],\"packageUris\":[\"http://schema.mathworks.com/mf0/Connector/R2020b\"],\"version\":\"1.0\"}"
  mabc : Outport
  Pmeas : Outport  Port=2
  Qmeas : Outport  Port=3
  tag scope: angle=global
  wires:
  VoltageCurrentControl/1(mabc) -> mabc/1
  Pref/1 -> Power Control/1(Pref)
  Qref/1 -> Power Control/3(Qref)
  Vgabc/1 -> Measurement/1(Vgabcc)
  Igabc/1 -> Measurement/2(Igabc)
  [angle] -> Measurement/3(Angle)
  Measurement/2(Pmeas) -> Pmeas/1
  Measurement/3(Qmeas) -> Qmeas/1
  Measurement/1(measure) -> VoltageCurrentControl/3(measure), Current Limiting/1(measure), Power Control/2(measure)
  Power Control/3(angle) -> [angle]
  Power Control/1(reactiveControl) -> Current Limiting/2(reactiveControl)
  Power Control/2(activeControl) -> VoltageCurrentControl/2(activeControl)
  Current Limiting/1(currentLimiting) -> VoltageCurrentControl/1(currentLimiting)

== system BatteryStoragePVPlantGFM/BESS & PV PARK/60 MWhr Battery Energy Storage/Variant Subsystem/Grid Following Support/Battery Inverter/GFL Battery Controller/Reference Current/Current limits ==
  Imax : Inport
  iqref : Inport  Port=2
  idref : Inport  Port=3
  Constant8 : Constant  Value=0
  Constant9 : Constant  Value=0
  Sqrt : Sqrt
  Sqrt1 : Sqrt
  Square{1..4} (4 alike) : Math  Operator=square
  Step2 : Step  Time=0.01  SampleTime=Ts
  Step3 : Step  Time=0.01  SampleTime=Ts
  Sum6 : Sum  Inputs=|+-
  Sum9 : Sum  Inputs=|+-
  Switch1 : Switch  Threshold=.01  SaturateOnIntegerOverflow=off  InputSameDT=off
  Switch2 : Switch  Threshold=.01  SaturateOnIntegerOverflow=off  InputSameDT=off
  iubd : Outport
  iubq : Outport  Port=2
  wires:
  Sum9/1 -> Switch2/1
  Step3/1 -> Switch2/2
  Step2/1 -> Switch1/2
  Switch2/1 -> Sqrt1/1
  Square1/1 -> Sum6/1
  Switch1/1 -> Sqrt/1
  iqref/1 -> Square2/1
  Square3/1 -> Sum9/1
  Sum6/1 -> Switch1/1
  Square2/1 -> Sum6/2
  Constant8/1 -> Switch1/3
  Square4/1 -> Sum9/2
  Constant9/1 -> Switch2/3
  Sqrt/1 -> iubd/1
  Imax/1 -> Square3/1, Square1/1
  Sqrt1/1 -> iubq/1
  idref/1 -> Square4/1

== system BatteryStoragePVPlantGFM/BESS & PV PARK/60 MWhr Battery Energy Storage/Variant Subsystem/Grid Following Support/Battery Inverter/GFL Battery Controller/Reference Current/Refernce id generation ==
  V_mag : Inport
  del f : Inport  Port=2
  ubid : Inport  Port=3
  Divide : Product  Inputs=/*
  Gain6 : Gain  Gain=-1
  P/Q Priority : Switch  Criteria=u2 ~= 0  SaturateOnIntegerOverflow=off  InputSameDT=off
  PU : Gain  Gain=1/(1*Base.MVA_base_new)
  P_ref : Constant  Value=GFLBatteryController.P_ref
  Priority Mode : Constant  Value=GFLBatteryController.Priority
  Saturation Dynamic2 : simulink/Discontinuities/Saturation Dynamic  OutMin=[]  OutMax=[]  OutDataTypeStr=Inherit: Same as second input  OutDataType=fixdt(1, 16)  OutScaling=2^-10  DoSatur=off
  Saturation1 : Saturate  UpperLimit=PVInverter.I_max_pu  LowerLimit=-PVInverter.I_max_pu
  Sum : Sum  Inputs=|++
  droop m_p : Gain  Gain=GFLBatteryController.m_p/(1*Base.MVA_base_new)
  ubid1 : InportShadow  Port=3
  id_ref : Outport
  wires:
  P_ref/1 -> PU/1
  droop m_p/1 -> Sum/1
  Sum/1 -> Divide/2
  ubid/1 -> Saturation Dynamic2/1
  Gain6/1 -> Saturation Dynamic2/3
  Saturation Dynamic2/1 -> P/Q Priority/3
  PU/1 -> Sum/2
  Priority Mode/1 -> P/Q Priority/2
  Saturation1/1 -> P/Q Priority/1
  ubid1/1 -> Gain6/1
  P/Q Priority/1 -> id_ref/1
  V_mag/1 -> Divide/1
  Divide/1 -> Saturation1/1, Saturation Dynamic2/2
  del f/1 -> droop m_p/1

== system BatteryStoragePVPlantGFM/BESS & PV PARK/60 MWhr Battery Energy Storage/Variant Subsystem/Grid Following Support/Battery Inverter/GFL Battery Controller/Reference Current/Refernce iq generation ==
  V_ref : Inport
  V_mag : Inport  Port=2
  LVRT_iq : Inport  Port=3
  ubiq : Inport  Port=4
  Q_ref : Inport  Port=5
  Divide1 : Product  Inputs=*/
  Gain1 : Gain  Gain=-1
  Gain7 : Gain  Gain=-1
  LVRT Priority : Switch  Threshold=.9  SaturateOnIntegerOverflow=off  InputSameDT=off
  P/Q Priority : Switch  Criteria=u2 ~= 0  SaturateOnIntegerOverflow=off  InputSameDT=off
  PU : Gain  Gain=1/(1*Base.MVA_base_new)
  Priority Mode : Constant  Value=GFLBatteryController.Priority
  Saturation Dynamic : simulink/Discontinuities/Saturation Dynamic  OutMin=[]  OutMax=[]  OutDataTypeStr=Inherit: Same as second input  OutDataType=fixdt(1, 16)  OutScaling=2^-10  DoSatur=off
  Saturation2 : Saturate  UpperLimit=1  LowerLimit=-1
  Saturation3 : Saturate  UpperLimit=PVInverter.I_max_pu  LowerLimit=-PVInverter.I_max_pu
  Sum : Sum  Inputs=|++
  Sum1 : Sum  Inputs=|-+
  droop m_v : Gain  Gain=GFLBatteryController.m_v
  ubiq1 : InportShadow  Port=4
  iq_ref : Outport
  wires:
  LVRT Priority/1 -> iq_ref/1
  Sum1/1 -> droop m_v/1
  P/Q Priority/1 -> LVRT Priority/1
  Gain1/1 -> LVRT Priority/3
  ubiq/1 -> Saturation Dynamic/1
  Saturation2/1 -> Gain1/1
  Saturation3/1 -> P/Q Priority/3
  Priority Mode/1 -> P/Q Priority/2
  Divide1/1 -> Saturation Dynamic/2, Saturation3/1
  Saturation Dynamic/1 -> P/Q Priority/1
  Gain7/1 -> Saturation Dynamic/3
  V_ref/1 -> Sum1/1
  LVRT_iq/1 -> Saturation2/1
  V_mag/1 -> Sum1/2, LVRT Priority/2, Divide1/2
  ubiq1/1 -> Gain7/1
  droop m_v/1 -> Sum/2
  Sum/1 -> Divide1/1
  Q_ref/1 -> PU/1
  PU/1 -> Sum/1
